simulink model "Regelkreis_PI"  (R2021a)
settings: Solver=ode45  StartTime=0.0  StopTime=0.75  MaxStep=0.0001  RelTol=1e-3  EnableMultiTasking=on
libraries: Regler x3
settings Model: Creator=zimmerma  LastModifiedBy=Manoli
settings SolverCC: AlgebraicLoopSolver=TrustRegion
settings DataIOCC: LimitDataPoints=on  SaveFormat=Array  SignalLoggingSaveFormat=ModelDataLogs  ReturnWorkspaceOutputs=off
settings OptimizationCC: ExpressionDepthLimit=2147483647  InitFltsAndDblsToZero=on  LifeSpan=inf
settings DebuggingCC: SaveWithParameterizedLinksMsg=none  UnderspecifiedInitializationDetection=Classic  MergeDetectMultiDrivingBlocksExec=none  SignalResolutionControl=TryResolveAllWithWarning  MultiTaskDSMMsg=warning  MultiTaskCondExecSysMsg=none  AllowSymbolicDim=off  StateNameClashWarn=warning  SFUnexpectedBacktrackingDiag=warning  SFNoUnconditionalDefaultTransitionDiag=warning  SFExecutionAtInitializationDiag=none  SFMachineParentedDataDiag=warning  ArithmeticOperatorsInVariantConditions=warning
settings HardwareCC: ProdBitPerPointer=32  ProdBitPerSizeT=32  ProdBitPerPtrDiffT=32  ProdLargestAtomicFloat=None  ProdIntDivRoundTo=Undefined  ProdEndianess=Unspecified  ProdWordSize=32  ProdHWDeviceType=32-bit Generic  TargetUnknown=on
settings ModelReferenceCC: PropagateSignalLabelsOutOfModel=off
settings SFSimCC: SimUseLocalCustomCode=off  CustomCodeUndefinedFunction=UseInterfaceOnly
settings RTWCC: RTWUseLocalCustomCode=off
settings CodeAppCC: StateflowObjectComments=on
settings GRTTargetCC: TargetFcnLib=ansi_tfl_tmw.mat  TargetLangStandard=C89/C90 (ANSI)  CombineOutputUpdateFcns=off  GRTInterface=on
settings ConfigComp: CovMetricSettings=dw  CovSaveCumulativeToWorkspaceVar=on  CovSaveSingleToWorkspaceVar=on  CovExternalEMLEnable=off

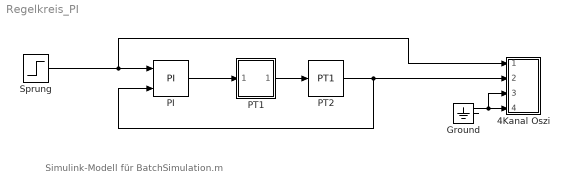
== system Regelkreis_PI ==
  note: Simulink-Modell für BatchSimulation.m
  4Kanal Oszi : Subsystem  mask(Oszilloskop){N=20000, k=[1 1 1 1], y=[-5 5], tmax=1}
      mask prompts: N "maximale Anzahl der Abtastpunkte N:"; k "Kanalverstaerkungen:"; y "[ymin ymax]:"
      mask help:
      | 4 Kanal Oszilloskop
      | Kanal1:rot    Kanal2:blau
      | Kanal3:grün Kanal4:magenta
      |
      | Achtung: Wenn das 4 Kanal Oszilloskop mehrfach in einem Blockschaltbild
      | verwendet  wird, müssen die Bezeichnungen der Variablen x1, ..., x4 und t in
      | den Simulink->Matlab Blöcken geändert werden (Edit - Look under Mask),
      | sonst überschreiben die Signale eines Oszilloskops die Werte des anderen
      | Oszilloskops im Matlab-Workspace.
      mask Help: 4 Kanal Oszilloskop mit automat. Skalierung\nKanalverstärkung einstellbar\nKanal1:rot, Kanal2:blau\nKanal3:grün, Kanal4:magenta
      mask Display: disp('Oszi')
  Ground : Ground
  PI : Regler/PI  kp=kp  Tn=Tn
  PT1 : Subsystem  mask(PT1){k=4, T1=10 / 1000}
      mask prompts: k "Verstärkung kp"; T1 "Zeitkonstante T1"
      mask help: PT1-Glied kp/(1+s·T1)
      mask Help: PT1 Tiefpaß 1.Ordnung mit Verstärkung kp und Zeitkonstante T1
      mask Display: disp('PT1')
  PT2 : Regler/PT1  k=1  T1=100 / 1000
  Sprung : Step  Time=0.000001  SampleTime=0
  wires:
  Sprung/1 -> PI/1, 4Kanal Oszi/1(in_1)
  PI/1 -> PT1/1(In1)
  PT1/1(Out1) -> PT2/1
  Ground/1 -> 4Kanal Oszi/3(in_3), 4Kanal Oszi/4(in_4)
  PT2/1 -> PI/2, 4Kanal Oszi/2(in_2)

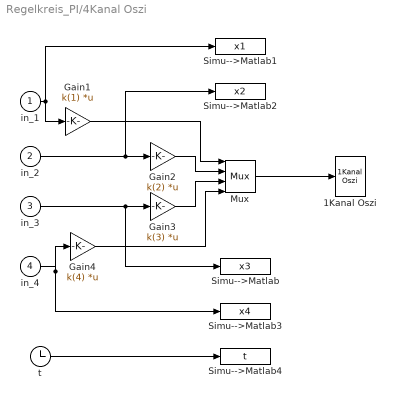
== system Regelkreis_PI/4Kanal Oszi ==
  in_1 : Inport
  in_2 : Inport  Port=2
  in_3 : Inport  Port=3
  in_4 : Inport  Port=4
  1Kanal Oszi : Regler/1Kanal Oszi  TR=1  ymin=0  ymax=1  npts=1024  color='r-/b-/g-/m-'
  Gain1 : Gain  Gain=k(1)  Multiplication=Matrix(K*u)  SaturateOnIntegerOverflow=on  OutDataTypeStr=Inherit: Same as input  ParamDataTypeStr=Inherit: Same as input
  Gain2 : Gain  Gain=k(2)  Multiplication=Matrix(K*u)  SaturateOnIntegerOverflow=on  OutDataTypeStr=Inherit: Same as input  ParamDataTypeStr=Inherit: Same as input
  Gain3 : Gain  Gain=k(3)  Multiplication=Matrix(K*u)  SaturateOnIntegerOverflow=on  OutDataTypeStr=Inherit: Same as input  ParamDataTypeStr=Inherit: Same as input
  Gain4 : Gain  Gain=k(4)  Multiplication=Matrix(K*u)  SaturateOnIntegerOverflow=on  OutDataTypeStr=Inherit: Same as input  ParamDataTypeStr=Inherit: Same as input
  Mux : Mux
  Simu-->Matlab : ToWorkspace  VariableName=x3
      settings: MaxDataPoints=N
  Simu-->Matlab1 : ToWorkspace  VariableName=x1
      settings: MaxDataPoints=N
  Simu-->Matlab2 : ToWorkspace  VariableName=x2
      settings: MaxDataPoints=N
  Simu-->Matlab3 : ToWorkspace  VariableName=x4
      settings: MaxDataPoints=N
  Simu-->Matlab4 : ToWorkspace  VariableName=t
      settings: MaxDataPoints=N
  t : Clock
  wires:
  t/1 -> Simu-->Matlab4/1
  Mux/1 -> 1Kanal Oszi/1
  in_2/1 -> Simu-->Matlab2/1, Gain2/1
  in_3/1 -> Simu-->Matlab/1, Gain3/1
  Gain2/1 -> Mux/2
  Gain3/1 -> Mux/3
  in_4/1 -> Simu-->Matlab3/1, Gain4/1
  Gain4/1 -> Mux/4
  Gain1/1 -> Mux/1
  in_1/1 -> Simu-->Matlab1/1, Gain1/1

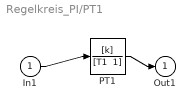
== system Regelkreis_PI/PT1 ==
  In1 : Inport
  PT1 : TransferFcn  Numerator=[k]  Denominator="[T1  1]"
  Out1 : Outport  VectorParamsAs1DForOutWhenUnconnected=off
  wires:
  PT1/1 -> Out1/1
  In1/1 -> PT1/1
